simulink subsystem "normalizePWM_sub"  (R2024a)
settings: Solver=VariableStepAuto  StartTime=0.0  StopTime=10.0  RelTol=1e-3
settings Model: Creator=UASG  LastModifiedBy=UASG

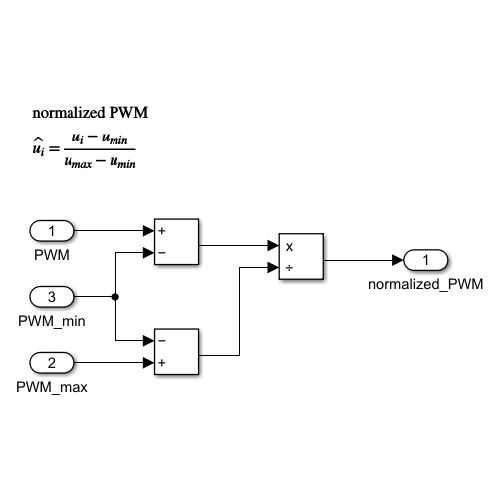
[thumbnail: Simulink's stored preview of the top-level diagram]
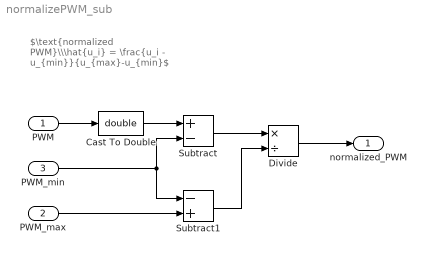
== system normalizePWM_sub ==
  note: $\text{normalized PWM}\\\hat{u_i} = \frac{u_i - u_{min}}{u_{max}-u_{min}$
  PWM : Inport
  PWM_max : Inport  Port=2
  PWM_min : Inport  Port=3
  Cast To Double : DataTypeConversion  OutDataTypeStr=double  SaturateOnIntegerOverflow=off  RndMeth=Floor
  Divide : Product  Inputs=*/
  Subtract : Sum  Inputs=+-
  Subtract1 : Sum  Inputs=-+
  normalized_PWM : Outport
  wires:
  PWM/1 -> Cast To Double/1
  PWM_min/1 -> Subtract1/1, Subtract/2
  PWM_max/1 -> Subtract1/2
  Subtract/1 -> Divide/1
  Subtract1/1 -> Divide/2
  Divide/1 -> normalized_PWM/1
  Cast To Double/1 -> Subtract/1
